simulink model "PWMGenerator"  (R2018b)
settings: Solver=VariableStepAuto  StartTime=0.0  StopTime=50000  RelTol=1e-3
libraries: hdlsllib x15, simulink x5
settings Model: Creator=wachala.j  LastModifiedBy=vttre
settings SFSimCC: SimUseLocalCustomCode=off
settings RTWCC: RTWUseLocalCustomCode=off
settings CodeAppCC: StateflowObjectComments=on

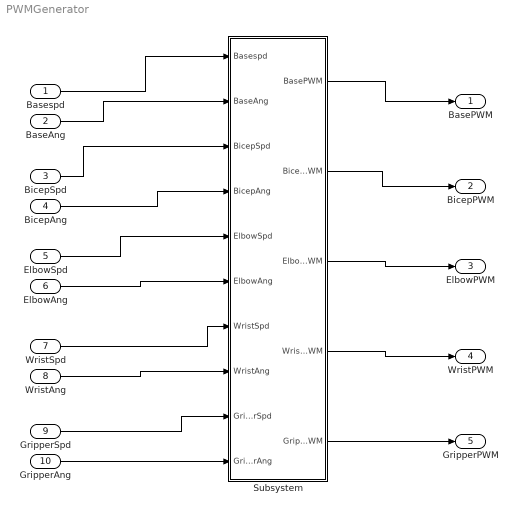
== system PWMGenerator ==
  Basespd : Inport
  BaseAng : Inport  Port=2
  BicepSpd : Inport  Port=3
  BicepAng : Inport  Port=4
  ElbowSpd : Inport  Port=5
  ElbowAng : Inport  Port=6
  WristSpd : Inport  Port=7
  WristAng : Inport  Port=8
  GripperSpd : Inport  Port=9
  GripperAng : Inport  Port=10
  Subsystem : Subsystem
  BasePWM : Outport
  BicepPWM : Outport  Port=2
  ElbowPWM : Outport  Port=3
  WristPWM : Outport  Port=4
  GripperPWM : Outport  Port=5
  wires:
  Basespd/1 -> Subsystem/1(Basespd)
  BaseAng/1 -> Subsystem/2(BaseAng)
  BicepSpd/1 -> Subsystem/3(BicepSpd)
  BicepAng/1 -> Subsystem/4(BicepAng)
  ElbowSpd/1 -> Subsystem/5(ElbowSpd)
  ElbowAng/1 -> Subsystem/6(ElbowAng)
  WristSpd/1 -> Subsystem/7(WristSpd)
  WristAng/1 -> Subsystem/8(WristAng)
  GripperSpd/1 -> Subsystem/9(GripperSpd)
  GripperAng/1 -> Subsystem/10(GripperAng)
  Subsystem/1(BasePWM) -> BasePWM/1
  Subsystem/2(BicepPWM) -> BicepPWM/1
  Subsystem/3(ElbowPWM) -> ElbowPWM/1
  Subsystem/4(WristPWM) -> WristPWM/1
  Subsystem/5(GripperPWM) -> GripperPWM/1

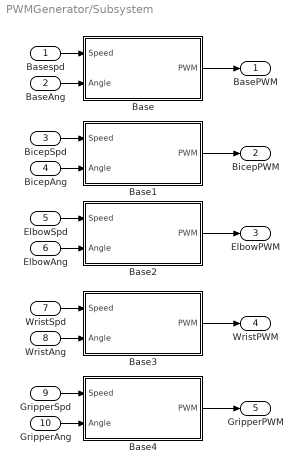
== system PWMGenerator/Subsystem ==
  Basespd : Inport
  BaseAng : Inport  Port=2
  BicepSpd : Inport  Port=3
  BicepAng : Inport  Port=4
  ElbowSpd : Inport  Port=5
  ElbowAng : Inport  Port=6
  WristSpd : Inport  Port=7
  WristAng : Inport  Port=8
  GripperSpd : Inport  Port=9
  GripperAng : Inport  Port=10
  Base : Subsystem
  Base1 : Subsystem
  Base2 : Subsystem
  Base3 : Subsystem
  Base4 : Subsystem
  BasePWM : Outport
  BicepPWM : Outport  Port=2
  ElbowPWM : Outport  Port=3
  WristPWM : Outport  Port=4
  GripperPWM : Outport  Port=5
  wires:
  GripperSpd/1 -> Base4/1(Speed)
  BaseAng/1 -> Base/2(Angle)
  Base3/1(PWM) -> WristPWM/1
  BicepAng/1 -> Base1/2(Angle)
  WristAng/1 -> Base3/2(Angle)
  GripperAng/1 -> Base4/2(Angle)
  ElbowSpd/1 -> Base2/1(Speed)
  Base4/1(PWM) -> GripperPWM/1
  WristSpd/1 -> Base3/1(Speed)
  ElbowAng/1 -> Base2/2(Angle)
  Base2/1(PWM) -> ElbowPWM/1
  Base1/1(PWM) -> BicepPWM/1
  BicepSpd/1 -> Base1/1(Speed)
  Basespd/1 -> Base/1(Speed)
  Base/1(PWM) -> BasePWM/1

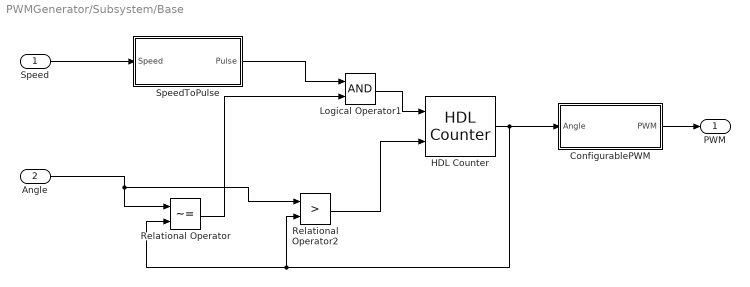
== system PWMGenerator/Subsystem/Base ==
  Speed : Inport
  Angle : Inport  Port=2
  ConfigurablePWM : Subsystem
  HDL Counter : hdlsllib/Sources/HDL Counter  CountType=Count limited  CountInit=90  CountStep=1  CountMax=180  CountFromType=Initial value  CountFrom=90  CountResetPort=off  CountLoadPort=off  CountEnbPort=on  CountDirPort=on  CountDataType=Unsigned  CountWordLen=8  CountFracLen=0  CountSampTime=1
      settings: SourceProductBaseCode=HD
  Logical Operator1 : Logic  AllPortsSameDT=off  OutDataTypeStr=boolean
  Relational Operator : RelationalOperator  Operator=~=  OutDataTypeStr=boolean  RndMeth=Simplest
  Relational Operator2 : RelationalOperator  Operator=>  OutDataTypeStr=boolean  RndMeth=Simplest
  SpeedToPulse : Subsystem
  PWM : Outport
  wires:
  Relational Operator/1 -> Logical Operator1/2
  Relational Operator2/1 -> HDL Counter/2
  SpeedToPulse/1("Pulse ") -> Logical Operator1/1
  ConfigurablePWM/1(PWM) -> PWM/1
  Angle/1 -> Relational Operator2/1, Relational Operator/1
  Speed/1 -> SpeedToPulse/1(Speed)
  HDL Counter/1 -> ConfigurablePWM/1(Angle), Relational Operator2/2, Relational Operator/2
  Logical Operator1/1 -> HDL Counter/1

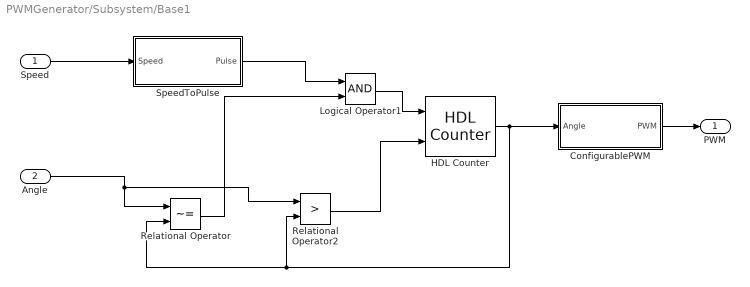
== system PWMGenerator/Subsystem/Base1 ==
  Speed : Inport
  Angle : Inport  Port=2
  ConfigurablePWM : Subsystem
  HDL Counter : hdlsllib/Sources/HDL Counter  CountType=Count limited  CountInit=90  CountStep=1  CountMax=180  CountFromType=Initial value  CountFrom=90  CountResetPort=off  CountLoadPort=off  CountEnbPort=on  CountDirPort=on  CountDataType=Unsigned  CountWordLen=8  CountFracLen=0  CountSampTime=1
      settings: SourceProductBaseCode=HD
  Logical Operator1 : Logic  AllPortsSameDT=off  OutDataTypeStr=boolean
  Relational Operator : RelationalOperator  Operator=~=  OutDataTypeStr=boolean  RndMeth=Simplest
  Relational Operator2 : RelationalOperator  Operator=>  OutDataTypeStr=boolean  RndMeth=Simplest
  SpeedToPulse : Subsystem
  PWM : Outport
  wires:
  Relational Operator/1 -> Logical Operator1/2
  Relational Operator2/1 -> HDL Counter/2
  SpeedToPulse/1("Pulse ") -> Logical Operator1/1
  ConfigurablePWM/1(PWM) -> PWM/1
  Angle/1 -> Relational Operator2/1, Relational Operator/1
  Speed/1 -> SpeedToPulse/1(Speed)
  HDL Counter/1 -> ConfigurablePWM/1(Angle), Relational Operator2/2, Relational Operator/2
  Logical Operator1/1 -> HDL Counter/1

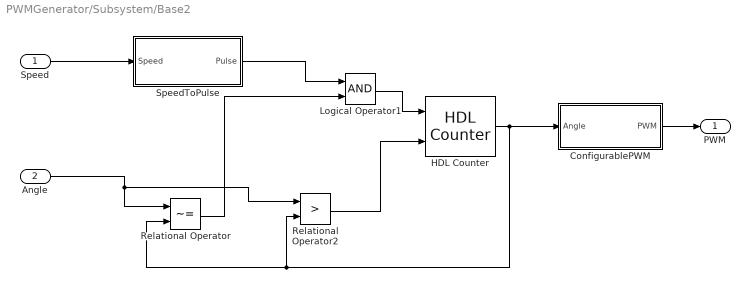
== system PWMGenerator/Subsystem/Base2 ==
  Speed : Inport
  Angle : Inport  Port=2
  ConfigurablePWM : Subsystem
  HDL Counter : hdlsllib/Sources/HDL Counter  CountType=Count limited  CountInit=90  CountStep=1  CountMax=180  CountFromType=Initial value  CountFrom=90  CountResetPort=off  CountLoadPort=off  CountEnbPort=on  CountDirPort=on  CountDataType=Unsigned  CountWordLen=8  CountFracLen=0  CountSampTime=1
      settings: SourceProductBaseCode=HD
  Logical Operator1 : Logic  AllPortsSameDT=off  OutDataTypeStr=boolean
  Relational Operator : RelationalOperator  Operator=~=  OutDataTypeStr=boolean  RndMeth=Simplest
  Relational Operator2 : RelationalOperator  Operator=>  OutDataTypeStr=boolean  RndMeth=Simplest
  SpeedToPulse : Subsystem
  PWM : Outport
  wires:
  Relational Operator/1 -> Logical Operator1/2
  Relational Operator2/1 -> HDL Counter/2
  SpeedToPulse/1("Pulse ") -> Logical Operator1/1
  ConfigurablePWM/1(PWM) -> PWM/1
  Angle/1 -> Relational Operator2/1, Relational Operator/1
  Speed/1 -> SpeedToPulse/1(Speed)
  HDL Counter/1 -> ConfigurablePWM/1(Angle), Relational Operator2/2, Relational Operator/2
  Logical Operator1/1 -> HDL Counter/1

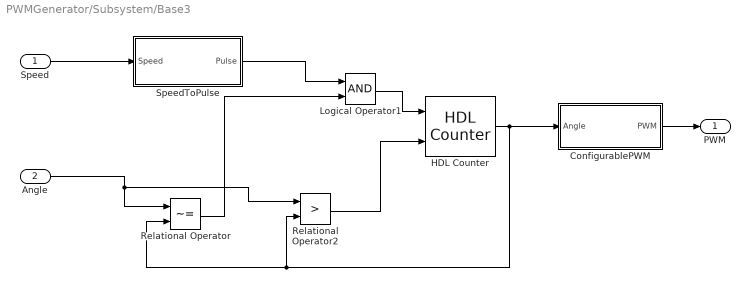
== system PWMGenerator/Subsystem/Base3 ==
  Speed : Inport
  Angle : Inport  Port=2
  ConfigurablePWM : Subsystem
  HDL Counter : hdlsllib/Sources/HDL Counter  CountType=Count limited  CountInit=90  CountStep=1  CountMax=180  CountFromType=Initial value  CountFrom=90  CountResetPort=off  CountLoadPort=off  CountEnbPort=on  CountDirPort=on  CountDataType=Unsigned  CountWordLen=8  CountFracLen=0  CountSampTime=1
      settings: SourceProductBaseCode=HD
  Logical Operator1 : Logic  AllPortsSameDT=off  OutDataTypeStr=boolean
  Relational Operator : RelationalOperator  Operator=~=  OutDataTypeStr=boolean  RndMeth=Simplest
  Relational Operator2 : RelationalOperator  Operator=>  OutDataTypeStr=boolean  RndMeth=Simplest
  SpeedToPulse : Subsystem
  PWM : Outport
  wires:
  Relational Operator/1 -> Logical Operator1/2
  Relational Operator2/1 -> HDL Counter/2
  SpeedToPulse/1("Pulse ") -> Logical Operator1/1
  ConfigurablePWM/1(PWM) -> PWM/1
  Angle/1 -> Relational Operator2/1, Relational Operator/1
  Speed/1 -> SpeedToPulse/1(Speed)
  HDL Counter/1 -> ConfigurablePWM/1(Angle), Relational Operator2/2, Relational Operator/2
  Logical Operator1/1 -> HDL Counter/1

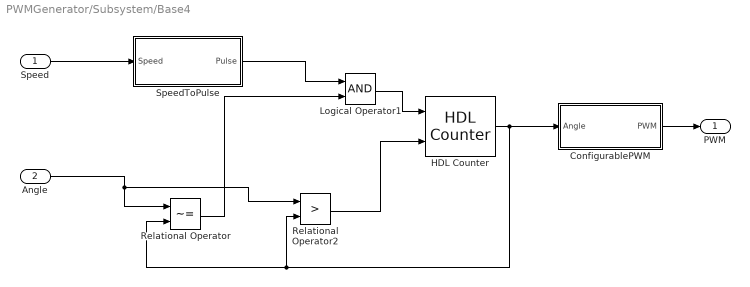
== system PWMGenerator/Subsystem/Base4 ==
  Speed : Inport
  Angle : Inport  Port=2
  ConfigurablePWM : Subsystem
  HDL Counter : hdlsllib/Sources/HDL Counter  CountType=Count limited  CountInit=90  CountStep=1  CountMax=180  CountFromType=Initial value  CountFrom=90  CountResetPort=off  CountLoadPort=off  CountEnbPort=on  CountDirPort=on  CountDataType=Unsigned  CountWordLen=8  CountFracLen=0  CountSampTime=1
      settings: SourceProductBaseCode=HD
  Logical Operator1 : Logic  AllPortsSameDT=off  OutDataTypeStr=boolean
  Relational Operator : RelationalOperator  Operator=~=  OutDataTypeStr=boolean  RndMeth=Simplest
  Relational Operator2 : RelationalOperator  Operator=>  OutDataTypeStr=boolean  RndMeth=Simplest
  SpeedToPulse : Subsystem
  PWM : Outport
  wires:
  Relational Operator/1 -> Logical Operator1/2
  Relational Operator2/1 -> HDL Counter/2
  SpeedToPulse/1("Pulse ") -> Logical Operator1/1
  ConfigurablePWM/1(PWM) -> PWM/1
  Angle/1 -> Relational Operator2/1, Relational Operator/1
  Speed/1 -> SpeedToPulse/1(Speed)
  HDL Counter/1 -> ConfigurablePWM/1(Angle), Relational Operator2/2, Relational Operator/2
  Logical Operator1/1 -> HDL Counter/1

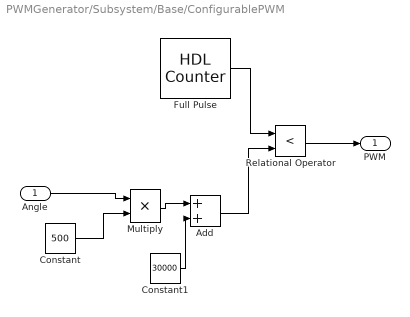
== system PWMGenerator/Subsystem/Base/ConfigurablePWM ==
  Angle : Inport  OutDataTypeStr=uint8
  Add : Sum
  Constant : Constant  Value=500  OutDataTypeStr=uint32  SampleTime=1
  Constant1 : Constant  Value=30000  OutDataTypeStr=uint32  SampleTime=1
  Full Pulse : hdlsllib/Sources/HDL Counter  CountType=Count limited  CountInit=0  CountStep=1  CountMax=1000000  CountFromType=Initial value  CountFrom=0  CountResetPort=off  CountLoadPort=off  CountEnbPort=off  CountDirPort=off  CountDataType=Unsigned  CountWordLen=32  CountFracLen=0  CountSampTime=1
      settings: SourceProductBaseCode=HD
  Multiply : Product  Inputs=**
  Relational Operator : RelationalOperator  Operator=<  OutDataTypeStr=boolean  RndMeth=Simplest
  PWM : Outport
  wires:
  Relational Operator/1 -> PWM/1
  Full Pulse/1 -> Relational Operator/1
  Angle/1 -> Multiply/1
  Multiply/1 -> Add/1
  Constant1/1 -> Add/2
  Add/1 -> Relational Operator/2
  Constant/1 -> Multiply/2

== system PWMGenerator/Subsystem/Base/SpeedToPulse ==
  Speed : Inport
  Compare To Constant : simulink/Logic and Bit Operations/Compare To Constant  relop===  const=0  OutDataTypeStr=boolean
  Constant1 : Constant  Value=50000000  OutDataTypeStr=uint32  SampleTime=1
  Divide : Product  Inputs=*/  SaturateOnIntegerOverflow=on  RndMeth=Zero
  HDL Counter : hdlsllib/Sources/HDL Counter  CountType=Free running  CountInit=0  CountStep=1  CountMax=25  CountFromType=Initial value  CountFrom=0  CountResetPort=on  CountLoadPort=off  CountEnbPort=off  CountDirPort=off  CountDataType=Unsigned  CountWordLen=32  CountFracLen=0  CountSampTime=1
      settings: SourceProductBaseCode=HD
  Relational Operator : RelationalOperator  Operator=<  OutDataTypeStr=boolean  RndMeth=Simplest
  "Pulse " : Outport
  wires:
  HDL Counter/1 -> Relational Operator/2, Compare To Constant/1
  Divide/1 -> Relational Operator/1
  Relational Operator/1 -> HDL Counter/1
  Compare To Constant/1 -> "Pulse "/1
  Speed/1 -> Divide/2
  Constant1/1 -> Divide/1

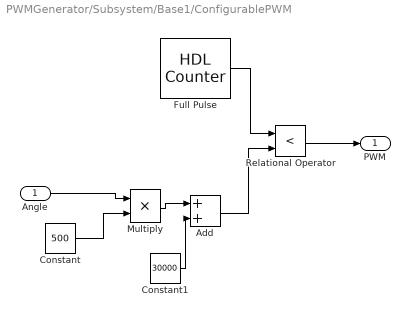
== system PWMGenerator/Subsystem/Base1/ConfigurablePWM ==
  Angle : Inport  OutDataTypeStr=uint8
  Add : Sum
  Constant : Constant  Value=500  OutDataTypeStr=uint32  SampleTime=1
  Constant1 : Constant  Value=30000  OutDataTypeStr=uint32  SampleTime=1
  Full Pulse : hdlsllib/Sources/HDL Counter  CountType=Count limited  CountInit=0  CountStep=1  CountMax=1000000  CountFromType=Initial value  CountFrom=0  CountResetPort=off  CountLoadPort=off  CountEnbPort=off  CountDirPort=off  CountDataType=Unsigned  CountWordLen=32  CountFracLen=0  CountSampTime=1
      settings: SourceProductBaseCode=HD
  Multiply : Product  Inputs=**
  Relational Operator : RelationalOperator  Operator=<  OutDataTypeStr=boolean  RndMeth=Simplest
  PWM : Outport
  wires:
  Relational Operator/1 -> PWM/1
  Full Pulse/1 -> Relational Operator/1
  Angle/1 -> Multiply/1
  Multiply/1 -> Add/1
  Constant1/1 -> Add/2
  Add/1 -> Relational Operator/2
  Constant/1 -> Multiply/2

== system PWMGenerator/Subsystem/Base1/SpeedToPulse ==
  Speed : Inport
  Compare To Constant : simulink/Logic and Bit Operations/Compare To Constant  relop===  const=0  OutDataTypeStr=boolean
  Constant1 : Constant  Value=50000000  OutDataTypeStr=uint32  SampleTime=1
  Divide : Product  Inputs=*/  SaturateOnIntegerOverflow=on  RndMeth=Zero
  HDL Counter : hdlsllib/Sources/HDL Counter  CountType=Free running  CountInit=0  CountStep=1  CountMax=25  CountFromType=Initial value  CountFrom=0  CountResetPort=on  CountLoadPort=off  CountEnbPort=off  CountDirPort=off  CountDataType=Unsigned  CountWordLen=32  CountFracLen=0  CountSampTime=1
      settings: SourceProductBaseCode=HD
  Relational Operator : RelationalOperator  Operator=<  OutDataTypeStr=boolean  RndMeth=Simplest
  "Pulse " : Outport
  wires:
  HDL Counter/1 -> Relational Operator/2, Compare To Constant/1
  Divide/1 -> Relational Operator/1
  Relational Operator/1 -> HDL Counter/1
  Compare To Constant/1 -> "Pulse "/1
  Speed/1 -> Divide/2
  Constant1/1 -> Divide/1

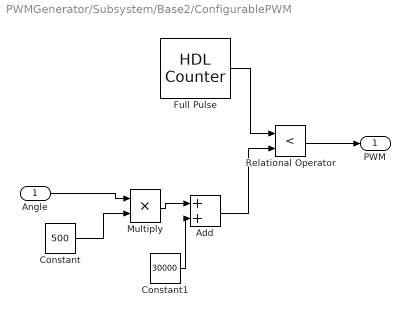
== system PWMGenerator/Subsystem/Base2/ConfigurablePWM ==
  Angle : Inport  OutDataTypeStr=uint8
  Add : Sum
  Constant : Constant  Value=500  OutDataTypeStr=uint32  SampleTime=1
  Constant1 : Constant  Value=30000  OutDataTypeStr=uint32  SampleTime=1
  Full Pulse : hdlsllib/Sources/HDL Counter  CountType=Count limited  CountInit=0  CountStep=1  CountMax=1000000  CountFromType=Initial value  CountFrom=0  CountResetPort=off  CountLoadPort=off  CountEnbPort=off  CountDirPort=off  CountDataType=Unsigned  CountWordLen=32  CountFracLen=0  CountSampTime=1
      settings: SourceProductBaseCode=HD
  Multiply : Product  Inputs=**
  Relational Operator : RelationalOperator  Operator=<  OutDataTypeStr=boolean  RndMeth=Simplest
  PWM : Outport
  wires:
  Relational Operator/1 -> PWM/1
  Full Pulse/1 -> Relational Operator/1
  Angle/1 -> Multiply/1
  Multiply/1 -> Add/1
  Constant1/1 -> Add/2
  Add/1 -> Relational Operator/2
  Constant/1 -> Multiply/2

== system PWMGenerator/Subsystem/Base2/SpeedToPulse ==
  Speed : Inport
  Compare To Constant : simulink/Logic and Bit Operations/Compare To Constant  relop===  const=0  OutDataTypeStr=boolean
  Constant1 : Constant  Value=50000000  OutDataTypeStr=uint32  SampleTime=1
  Divide : Product  Inputs=*/  SaturateOnIntegerOverflow=on  RndMeth=Zero
  HDL Counter : hdlsllib/Sources/HDL Counter  CountType=Free running  CountInit=0  CountStep=1  CountMax=25  CountFromType=Initial value  CountFrom=0  CountResetPort=on  CountLoadPort=off  CountEnbPort=off  CountDirPort=off  CountDataType=Unsigned  CountWordLen=32  CountFracLen=0  CountSampTime=1
      settings: SourceProductBaseCode=HD
  Relational Operator : RelationalOperator  Operator=<  OutDataTypeStr=boolean  RndMeth=Simplest
  "Pulse " : Outport
  wires:
  HDL Counter/1 -> Relational Operator/2, Compare To Constant/1
  Divide/1 -> Relational Operator/1
  Relational Operator/1 -> HDL Counter/1
  Compare To Constant/1 -> "Pulse "/1
  Speed/1 -> Divide/2
  Constant1/1 -> Divide/1

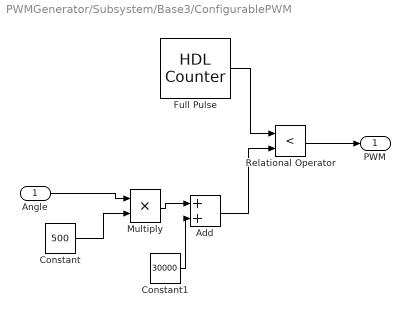
== system PWMGenerator/Subsystem/Base3/ConfigurablePWM ==
  Angle : Inport  OutDataTypeStr=uint8
  Add : Sum
  Constant : Constant  Value=500  OutDataTypeStr=uint32  SampleTime=1
  Constant1 : Constant  Value=30000  OutDataTypeStr=uint32  SampleTime=1
  Full Pulse : hdlsllib/Sources/HDL Counter  CountType=Count limited  CountInit=0  CountStep=1  CountMax=1000000  CountFromType=Initial value  CountFrom=0  CountResetPort=off  CountLoadPort=off  CountEnbPort=off  CountDirPort=off  CountDataType=Unsigned  CountWordLen=32  CountFracLen=0  CountSampTime=1
      settings: SourceProductBaseCode=HD
  Multiply : Product  Inputs=**
  Relational Operator : RelationalOperator  Operator=<  OutDataTypeStr=boolean  RndMeth=Simplest
  PWM : Outport
  wires:
  Relational Operator/1 -> PWM/1
  Full Pulse/1 -> Relational Operator/1
  Angle/1 -> Multiply/1
  Multiply/1 -> Add/1
  Constant1/1 -> Add/2
  Add/1 -> Relational Operator/2
  Constant/1 -> Multiply/2

== system PWMGenerator/Subsystem/Base3/SpeedToPulse ==
  Speed : Inport
  Compare To Constant : simulink/Logic and Bit Operations/Compare To Constant  relop===  const=0  OutDataTypeStr=boolean
  Constant1 : Constant  Value=50000000  OutDataTypeStr=uint32  SampleTime=1
  Divide : Product  Inputs=*/  SaturateOnIntegerOverflow=on  RndMeth=Zero
  HDL Counter : hdlsllib/Sources/HDL Counter  CountType=Free running  CountInit=0  CountStep=1  CountMax=25  CountFromType=Initial value  CountFrom=0  CountResetPort=on  CountLoadPort=off  CountEnbPort=off  CountDirPort=off  CountDataType=Unsigned  CountWordLen=32  CountFracLen=0  CountSampTime=1
      settings: SourceProductBaseCode=HD
  Relational Operator : RelationalOperator  Operator=<  OutDataTypeStr=boolean  RndMeth=Simplest
  "Pulse " : Outport
  wires:
  HDL Counter/1 -> Relational Operator/2, Compare To Constant/1
  Divide/1 -> Relational Operator/1
  Relational Operator/1 -> HDL Counter/1
  Compare To Constant/1 -> "Pulse "/1
  Speed/1 -> Divide/2
  Constant1/1 -> Divide/1

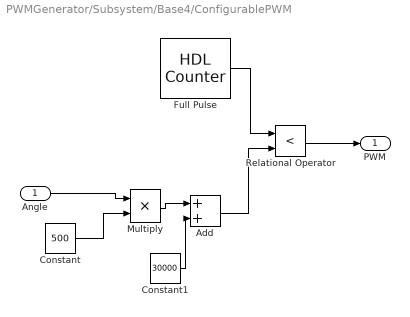
== system PWMGenerator/Subsystem/Base4/ConfigurablePWM ==
  Angle : Inport  OutDataTypeStr=uint8
  Add : Sum
  Constant : Constant  Value=500  OutDataTypeStr=uint32  SampleTime=1
  Constant1 : Constant  Value=30000  OutDataTypeStr=uint32  SampleTime=1
  Full Pulse : hdlsllib/Sources/HDL Counter  CountType=Count limited  CountInit=0  CountStep=1  CountMax=1000000  CountFromType=Initial value  CountFrom=0  CountResetPort=off  CountLoadPort=off  CountEnbPort=off  CountDirPort=off  CountDataType=Unsigned  CountWordLen=32  CountFracLen=0  CountSampTime=1
      settings: SourceProductBaseCode=HD
  Multiply : Product  Inputs=**
  Relational Operator : RelationalOperator  Operator=<  OutDataTypeStr=boolean  RndMeth=Simplest
  PWM : Outport
  wires:
  Relational Operator/1 -> PWM/1
  Full Pulse/1 -> Relational Operator/1
  Angle/1 -> Multiply/1
  Multiply/1 -> Add/1
  Constant1/1 -> Add/2
  Add/1 -> Relational Operator/2
  Constant/1 -> Multiply/2

== system PWMGenerator/Subsystem/Base4/SpeedToPulse ==
  Speed : Inport
  Compare To Constant : simulink/Logic and Bit Operations/Compare To Constant  relop===  const=0  OutDataTypeStr=boolean
  Constant1 : Constant  Value=50000000  OutDataTypeStr=uint32  SampleTime=1
  Divide : Product  Inputs=*/  SaturateOnIntegerOverflow=on  RndMeth=Zero
  HDL Counter : hdlsllib/Sources/HDL Counter  CountType=Free running  CountInit=0  CountStep=1  CountMax=25  CountFromType=Initial value  CountFrom=0  CountResetPort=on  CountLoadPort=off  CountEnbPort=off  CountDirPort=off  CountDataType=Unsigned  CountWordLen=32  CountFracLen=0  CountSampTime=1
      settings: SourceProductBaseCode=HD
  Relational Operator : RelationalOperator  Operator=<  OutDataTypeStr=boolean  RndMeth=Simplest
  "Pulse " : Outport
  wires:
  HDL Counter/1 -> Relational Operator/2, Compare To Constant/1
  Divide/1 -> Relational Operator/1
  Relational Operator/1 -> HDL Counter/1
  Compare To Constant/1 -> "Pulse "/1
  Speed/1 -> Divide/2
  Constant1/1 -> Divide/1
